simulink model "BB_DT_RRC_filters_EyeP_2020"  (R2020a)
settings: Solver=VariableStepDiscrete  StartTime=0.0  StopTime=L  RelTol=1e-3  AbsTol=1e-6  EnableMultiTasking=on
values from neighbouring files (symbols this model uses):
  G = 4    [ISI_init.m]
  N = 20    [ISI_init.m]
  R = 0.6    [ISI_init.m]
  T = 1e-3    (= 0.001)    [ISI_init.m]
undefined symbols (not defined in the file or in its folder): gcbh, rcfiltgaincompat
libraries: simulink_extras x9, commsequence2 x5, simulink x3, commfilt2 x2, commchan3 x1, dsparch4 x1
settings Model: Creator=calin  LastModifiedBy=Calin Vladeanu
settings DataIOCC: LimitDataPoints=on  SaveFormat=Array  SignalLoggingSaveFormat=ModelDataLogs  ReturnWorkspaceOutputs=off
settings OptimizationCC: InitFltsAndDblsToZero=on  LifeSpan=inf
settings DebuggingCC: SaveWithParameterizedLinksMsg=none  UnderspecifiedInitializationDetection=Classic  MergeDetectMultiDrivingBlocksExec=none  SignalResolutionControl=TryResolveAllWithWarning  SolverPrmCheckMsg=warning  MultiTaskDSMMsg=warning  MultiTaskCondExecSysMsg=none  FcnCallInpInsideContextMsg=warning  StateNameClashWarn=warning  SFUnexpectedBacktrackingDiag=warning  SFNoUnconditionalDefaultTransitionDiag=warning  SFExecutionAtInitializationDiag=none  ArithmeticOperatorsInVariantConditions=warning
settings HardwareCC: ProdBitPerPointer=32  ProdBitPerSizeT=32  ProdBitPerPtrDiffT=32  ProdLargestAtomicFloat=None  ProdIntDivRoundTo=Undefined  ProdEndianess=Unspecified  ProdWordSize=32  ProdHWDeviceType=32-bit Generic
settings ModelReferenceCC: PropagateSignalLabelsOutOfModel=off
settings SFSimCC: SimUseLocalCustomCode=off  CustomCodeUndefinedFunction=UseInterfaceOnly
settings RTWCC: RTWUseLocalCustomCode=off
settings CodeAppCC: StateflowObjectComments=on
settings GRTTargetCC: TargetFcnLib=ansi_tfl_tmw.mat  TargetLangStandard=C89/C90 (ANSI)  CombineOutputUpdateFcns=off  GRTInterface=on
settings ConfigComp: CovMetricSettings=dw  CovHtmlReporting=on  CovSaveCumulativeToWorkspaceVar=on  CovSaveSingleToWorkspaceVar=on  CovExternalEMLEnable=off

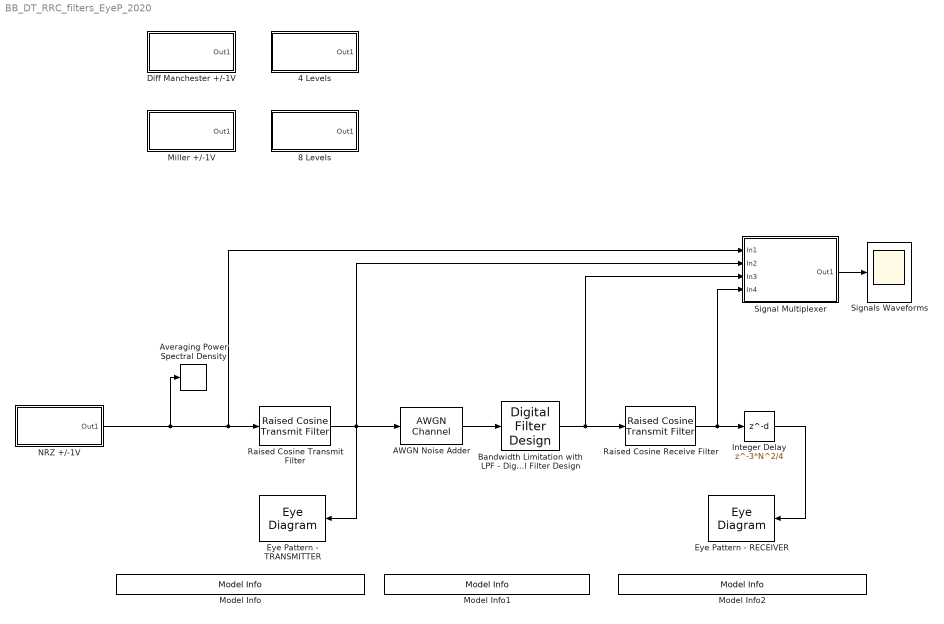
== system BB_DT_RRC_filters_EyeP_2020 ==
  4 Levels : Subsystem
  "8 Levels " : Subsystem
  AWGN Noise Adder : commchan3/AWGN Channel  InputProcessing=Columns as channels (frame based)  seed=67  noiseMode="Signal to noise ratio  (SNR)"  EbNodB=10  EsNodB=10  SNRdB=SNRdB  bitsPerSym=1  Ps=1  Tsym=1  variance=1
  Averaging Power Spectral Density : simulink_extras/Additional Sinks/Averaging Power Spectral Density  npts=512  fftpts=4096  HowOften=256  sampleT=T/8
      link override sfunpsd: FunctionName=sfunpsd_mod  Parameters=fftpts,npts,HowOften,offset,ts,1,type_disp
      settings: SourceProductBaseCode=SL
  Bandwidth Limitation with LPF - Digital Filter Design : dsparch4/Digital Filter Design  mwdsp_browser_bugfix_var=off
  Diff Manchester +/-1V : Subsystem
  Eye Pattern - RECEIVER : EyeDiagram  Tag=EyeDiagram
  Eye Pattern - TRANSMITTER : EyeDiagram  Tag=EyeDiagram
  Integer Delay : Delay  DelayLength=3*N^2/4
  Miller +/-1V : Subsystem
  Model Info : simulink/Model-Wide Utilities/Model Info  Frame=on  DisplayStringWithTags=TRANSMITTER  HorizontalTextAlignment=Center  LeftAlignmentValue=0.5
  Model Info1 : simulink/Model-Wide Utilities/Model Info  Frame=on  DisplayStringWithTags=CHANNEL MODEL  HorizontalTextAlignment=Center  LeftAlignmentValue=0.5
  Model Info2 : simulink/Model-Wide Utilities/Model Info  Frame=on  DisplayStringWithTags=RECEIVER  HorizontalTextAlignment=Center  LeftAlignmentValue=0.5
  NRZ +/-1V : Subsystem
  Raised Cosine Receive Filter : commfilt2/Raised Cosine Transmit Filter  filtType=Square root  R=R  filtSpan=2*(G)  N=N  filterGain=(sqrt(N))*rcfiltgaincompat(gcbh)  InputProcessing=Columns as channels (frame based)  RateOptions=Allow multirate processing  framing=Mute  checkCoeff=off  variableName=rcTxFilt1  checkGain=User-specified  sampMode=Mute  saveAsFlag=0  currentFiltSpan=2*(G)  D=G  launchFVT=off  roundingMode=Floor  overflowMode=off  coeffDataTypeStr=Inherit: Same word length as input  coeffMin=[]  coeffMax=[]  coeffLastDataTypeStr=Inherit: Same word length as input  outputDataTypeStr=Inherit: Same as accumulator  outputMin=[]  outputMax=[]  outputLastDataTypeStr=Inherit: Same as accumulator
  Raised Cosine Transmit Filter : commfilt2/Raised Cosine Transmit Filter  filtType=Square root  R=R  filtSpan=2*(G)  N=N  filterGain=(sqrt(N))*rcfiltgaincompat(gcbh)  InputProcessing=Columns as channels (frame based)  RateOptions=Allow multirate processing  framing=Mute  checkCoeff=off  variableName=rcTxFilt  checkGain=User-specified  sampMode=Mute  saveAsFlag=0  currentFiltSpan=2*(G)  D=G  launchFVT=off  roundingMode=Floor  overflowMode=off  coeffDataTypeStr=Inherit: Same word length as input  coeffMin=[]  coeffMax=[]  coeffLastDataTypeStr=Inherit: Same word length as input  outputDataTypeStr=Inherit: Same as accumulator  outputMin=[]  outputMax=[]  outputLastDataTypeStr=Inherit: Same as accumulator
  Signal Multiplexer : Subsystem
  Signals Waveforms : Scope
  wires:
  Raised Cosine Transmit Filter/1 -> AWGN Noise Adder/1, Eye Pattern - TRANSMITTER/1, Signal Multiplexer/2(In2)
  Raised Cosine Receive Filter/1 -> Integer Delay/1, Signal Multiplexer/4(In4)
  Bandwidth Limitation with LPF - Digital Filter Design/1 -> Raised Cosine Receive Filter/1, Signal Multiplexer/3(In3)
  AWGN Noise Adder/1 -> Bandwidth Limitation with LPF - Digital Filter Design/1
  Integer Delay/1 -> Eye Pattern - RECEIVER/1
  Signal Multiplexer/1(Out1) -> Signals Waveforms/1
  NRZ +/-1V/1(Out1) -> Averaging Power Spectral Density/1, Raised Cosine Transmit Filter/1, Signal Multiplexer/1(In1)

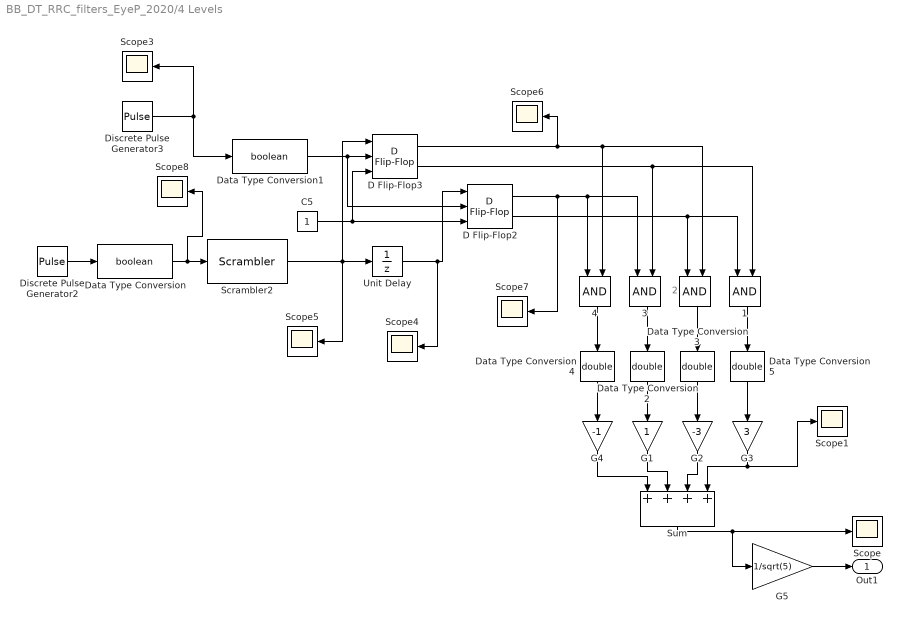
== system BB_DT_RRC_filters_EyeP_2020/4 Levels ==
  note: 2
  " " : Logic  OutDataTypeStr=boolean
  " 1" : Logic  OutDataTypeStr=boolean
  3 : Logic  OutDataTypeStr=boolean
  4 : Logic  OutDataTypeStr=boolean
  C5 : Constant
  D Flip-Flop2 : simulink_extras/Flip Flops/D Flip-Flop
  D Flip-Flop3 : simulink_extras/Flip Flops/D Flip-Flop
  Data Type Conversion : DataTypeConversion  OutDataTypeStr=boolean
  Data Type Conversion1 : DataTypeConversion  OutDataTypeStr=boolean
  Data Type Conversion{2..5} (4 alike) : DataTypeConversion  OutDataTypeStr=double
  Discrete Pulse Generator2 : DiscretePulseGenerator  Period=8  SampleTime=T
      settings: AttributesFormatString=1:7
  Discrete Pulse Generator3 : DiscretePulseGenerator  Period=4  PhaseDelay=2  SampleTime=T/2
      settings: AttributesFormatString=1:5
  G1 : Gain  OutDataTypeStr=double  SaturateOnIntegerOverflow=on  ParamDataTypeStr=Inherit: Same as input
  G2 : Gain  Gain=-3  OutDataTypeStr=double  SaturateOnIntegerOverflow=on  ParamDataTypeStr=Inherit: Same as input
  G3 : Gain  Gain=3  OutDataTypeStr=double  SaturateOnIntegerOverflow=on  ParamDataTypeStr=Inherit: Same as input
  G4 : Gain  Gain=-1  OutDataTypeStr=double  SaturateOnIntegerOverflow=on  ParamDataTypeStr=Inherit: Same as input
  G5 : Gain  Gain=1/sqrt(5)  OutDataTypeStr=double  SaturateOnIntegerOverflow=on  ParamDataTypeStr=Inherit: Same as input
  Scope{,1,3..8} (8 alike) : Scope
  Scrambler2 : commsequence2/Scrambler  M=2  poly=[0 -1 -7]  iniStaSource=Dialog Parameter  ini_sta=[1 1 1 1 1 1 1]  resetViaPort=off
      settings: SourceProductBaseCode=CM
  Sum : Sum  Inputs=++++  InputSameDT=on  AccumDataTypeStr=double  OutDataTypeStr=double  SaturateOnIntegerOverflow=on
  Unit Delay : UnitDelay  InitialCondition=1  SampleTime=-1  HasFrameUpgradeWarning=on
  Out1 : Outport  VectorParamsAs1DForOutWhenUnconnected=off
  wires:
  Sum/1 -> G5/1, Scope/1
  3/1 -> Data Type Conversion2/1
  " 1"/1 -> Data Type Conversion5/1
  D Flip-Flop2/1 -> 3/1, 4/1, Scope7/1
  D Flip-Flop2/2 -> " 1"/1, " "/1
  Scrambler2/1 -> D Flip-Flop3/1, Unit Delay/1, Scope5/1
  4/1 -> Data Type Conversion4/1
  C5/1 -> D Flip-Flop3/3, D Flip-Flop2/3
  Unit Delay/1 -> D Flip-Flop2/1, Scope4/1
  Discrete Pulse Generator2/1 -> Data Type Conversion/1
  D Flip-Flop3/1 -> " "/2, 4/2, Scope6/1
  " "/1 -> Data Type Conversion3/1
  D Flip-Flop3/2 -> " 1"/2, 3/2
  Discrete Pulse Generator3/1 -> Data Type Conversion1/1, Scope3/1
  Data Type Conversion/1 -> Scope8/1, Scrambler2/1
  Data Type Conversion1/1 -> D Flip-Flop3/2, D Flip-Flop2/2
  G4/1 -> Sum/1
  G1/1 -> Sum/2
  G2/1 -> Sum/3
  G3/1 -> Scope1/1, Sum/4
  Data Type Conversion4/1 -> G4/1
  Data Type Conversion2/1 -> G1/1
  Data Type Conversion3/1 -> G2/1
  Data Type Conversion5/1 -> G3/1
  G5/1 -> Out1/1

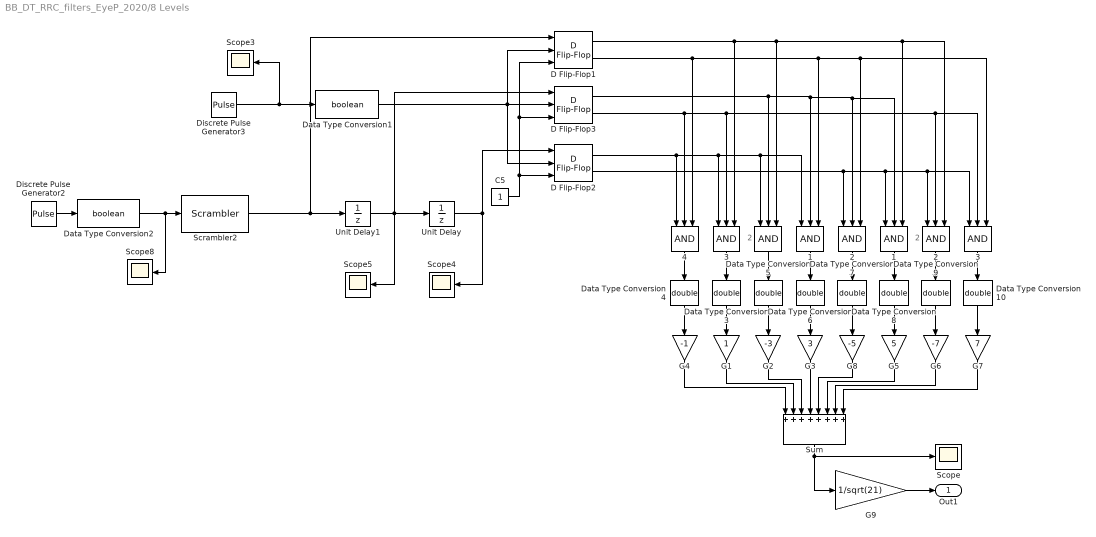
== system BB_DT_RRC_filters_EyeP_2020/8 Levels  ==
  note: 2
  note: 2
   {,1..3} (4 alike) : Logic  Inputs=3
  {1..4} (4 alike) : Logic  Inputs=3
  C5 : Constant
  D Flip-Flop1 : simulink_extras/Flip Flops/D Flip-Flop
  D Flip-Flop2 : simulink_extras/Flip Flops/D Flip-Flop
  D Flip-Flop3 : simulink_extras/Flip Flops/D Flip-Flop
  Data Type Conversion1 : DataTypeConversion  OutDataTypeStr=boolean
  Data Type Conversion{3..10} (8 alike) : DataTypeConversion  OutDataTypeStr=double
  Data Type Conversion2 : DataTypeConversion  OutDataTypeStr=boolean
  Discrete Pulse Generator2 : DiscretePulseGenerator  Period=8  SampleTime=2*pi/10000
      settings: AttributesFormatString=1:7
  Discrete Pulse Generator3 : DiscretePulseGenerator  Period=6  PhaseDelay=4  SampleTime=2*pi/20000
      settings: AttributesFormatString=1:5
  G1 : Gain  OutDataTypeStr=double  SaturateOnIntegerOverflow=on  ParamDataTypeStr=Inherit: Same as input
  G2 : Gain  Gain=-3  OutDataTypeStr=double  SaturateOnIntegerOverflow=on  ParamDataTypeStr=Inherit: Same as input
  G3 : Gain  Gain=3  OutDataTypeStr=double  SaturateOnIntegerOverflow=on  ParamDataTypeStr=Inherit: Same as input
  G4 : Gain  Gain=-1  OutDataTypeStr=double  SaturateOnIntegerOverflow=on  ParamDataTypeStr=Inherit: Same as input
  G5 : Gain  Gain=5  OutDataTypeStr=double  SaturateOnIntegerOverflow=on  ParamDataTypeStr=Inherit: Same as input
  G6 : Gain  Gain=-7  OutDataTypeStr=double  SaturateOnIntegerOverflow=on  ParamDataTypeStr=Inherit: Same as input
  G7 : Gain  Gain=7  OutDataTypeStr=double  SaturateOnIntegerOverflow=on  ParamDataTypeStr=Inherit: Same as input
  G8 : Gain  Gain=-5  OutDataTypeStr=double  SaturateOnIntegerOverflow=on  ParamDataTypeStr=Inherit: Same as input
  G9 : Gain  Gain=1/sqrt(21)  OutDataTypeStr=double  SaturateOnIntegerOverflow=on  ParamDataTypeStr=Inherit: Same as input
  Scope{,3..5,8} (5 alike) : Scope
  Scrambler2 : commsequence2/Scrambler  M=2  poly=[0 -1 -7]  iniStaSource=Dialog Parameter  ini_sta=[1 1 1 1 1 1 1]  resetViaPort=off
      settings: SourceProductBaseCode=CM
  Sum : Sum  Inputs=++++++++  InputSameDT=on  AccumDataTypeStr=double  OutDataTypeStr=double  SaturateOnIntegerOverflow=on
  Unit Delay : UnitDelay  InitialCondition=1  SampleTime=-1  HasFrameUpgradeWarning=on
  Unit Delay1 : UnitDelay  InitialCondition=1  SampleTime=-1  HasFrameUpgradeWarning=on
  Out1 : Outport  VectorParamsAs1DForOutWhenUnconnected=off
  wires:
  D Flip-Flop2/1 -> " 1"/1, " "/1, 3/1, 4/1
  D Flip-Flop3/1 -> 1/2, 2/2, " 1"/2, " "/2
  D Flip-Flop2/2 -> " 3"/1, " 2"/1, 1/1, 2/1
  G8/1 -> Sum/5
  " 2"/1 -> Data Type Conversion9/1
  G1/1 -> Sum/2
  D Flip-Flop1/2 -> " 3"/3, 2/3, " 1"/3, 4/3
  D Flip-Flop3/2 -> " 3"/2, " 2"/2, 3/2, 4/2
  " 1"/1 -> Data Type Conversion6/1
  " 3"/1 -> Data Type Conversion10/1
  3/1 -> Data Type Conversion3/1
  4/1 -> Data Type Conversion4/1
  " "/1 -> Data Type Conversion5/1
  G2/1 -> Sum/3
  2/1 -> Data Type Conversion7/1
  G7/1 -> Sum/8
  C5/1 -> D Flip-Flop1/3, D Flip-Flop3/3, D Flip-Flop2/3
  Discrete Pulse Generator2/1 -> Data Type Conversion2/1
  G3/1 -> Sum/4
  G6/1 -> Sum/7
  Unit Delay/1 -> D Flip-Flop2/1, Scope4/1
  G5/1 -> Sum/6
  Scrambler2/1 -> D Flip-Flop1/1, Unit Delay1/1
  G4/1 -> Sum/1
  D Flip-Flop1/1 -> " 2"/3, 1/3, " "/3, 3/3
  Unit Delay1/1 -> Unit Delay/1, Scope5/1, D Flip-Flop3/1
  Discrete Pulse Generator3/1 -> Data Type Conversion1/1, Scope3/1
  Sum/1 -> G9/1, Scope/1
  1/1 -> Data Type Conversion8/1
  Data Type Conversion1/1 -> D Flip-Flop2/2, D Flip-Flop3/2, D Flip-Flop1/2
  Data Type Conversion2/1 -> Scope8/1, Scrambler2/1
  Data Type Conversion4/1 -> G4/1
  Data Type Conversion3/1 -> G1/1
  Data Type Conversion5/1 -> G2/1
  Data Type Conversion6/1 -> G3/1
  Data Type Conversion7/1 -> G8/1
  Data Type Conversion8/1 -> G5/1
  Data Type Conversion9/1 -> G6/1
  Data Type Conversion10/1 -> G7/1
  G9/1 -> Out1/1

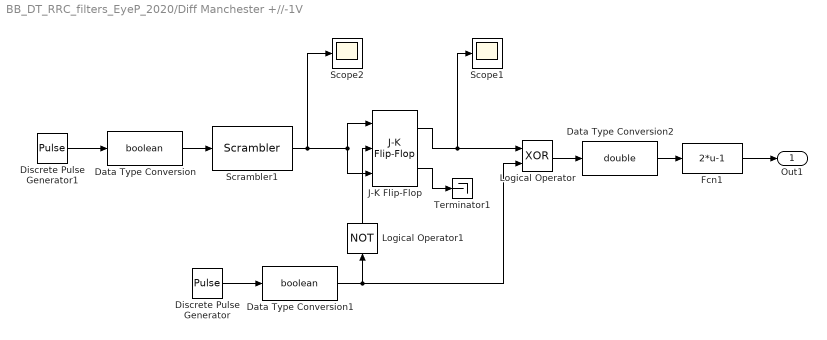
== system BB_DT_RRC_filters_EyeP_2020/Diff Manchester +//-1V ==
  Data Type Conversion : DataTypeConversion  OutDataTypeStr=boolean
  Data Type Conversion1 : DataTypeConversion  OutDataTypeStr=boolean
  Data Type Conversion2 : DataTypeConversion  OutDataTypeStr=double
  Discrete Pulse Generator : DiscretePulseGenerator  SampleTime=T/2
      settings: AttributesFormatString=CLK
  Discrete Pulse Generator1 : DiscretePulseGenerator  Period=8  SampleTime=T
      settings: AttributesFormatString=Data
  Fcn1 : Fcn  Expr=2*u-1
  J-K Flip-Flop : simulink_extras/Flip Flops/J-K Flip-Flop  initial_condition=0
  Logical Operator : Logic  Operator=XOR  OutDataTypeStr=boolean
  Logical Operator1 : Logic  Operator=NOT
  Scope1 : Scope
  Scope2 : Scope
  Scrambler1 : commsequence2/Scrambler  M=2  poly=[0 -1 -7]  iniStaSource=Dialog Parameter  ini_sta=[1 1 1 1 1 1 1]  resetViaPort=off
      settings: SourceProductBaseCode=CM
  Terminator1 : Terminator
  Out1 : Outport  VectorParamsAs1DForOutWhenUnconnected=off
  wires:
  Discrete Pulse Generator/1 -> Data Type Conversion1/1
  J-K Flip-Flop/2 -> Terminator1/1
  Logical Operator1/1 -> J-K Flip-Flop/2
  Scrambler1/1 -> Scope2/1, J-K Flip-Flop/1, J-K Flip-Flop/3
  Discrete Pulse Generator1/1 -> Data Type Conversion/1
  Logical Operator/1 -> Data Type Conversion2/1
  J-K Flip-Flop/1 -> Scope1/1, Logical Operator/1
  Data Type Conversion/1 -> Scrambler1/1
  Data Type Conversion1/1 -> Logical Operator1/1, Logical Operator/2
  Fcn1/1 -> Out1/1
  Data Type Conversion2/1 -> Fcn1/1

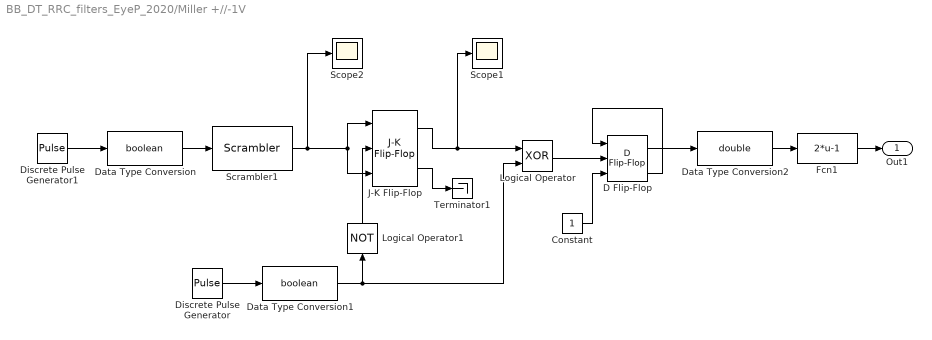
== system BB_DT_RRC_filters_EyeP_2020/Miller +//-1V ==
  Constant : Constant
  D Flip-Flop : simulink_extras/Flip Flops/D Flip-Flop
  Data Type Conversion : DataTypeConversion  OutDataTypeStr=boolean
  Data Type Conversion1 : DataTypeConversion  OutDataTypeStr=boolean
  Data Type Conversion2 : DataTypeConversion  OutDataTypeStr=double
  Discrete Pulse Generator : DiscretePulseGenerator  SampleTime=T/2
      settings: AttributesFormatString=CLK
  Discrete Pulse Generator1 : DiscretePulseGenerator  Period=8  SampleTime=T
      settings: AttributesFormatString=Data
  Fcn1 : Fcn  Expr=2*u-1
  J-K Flip-Flop : simulink_extras/Flip Flops/J-K Flip-Flop  initial_condition=0
  Logical Operator : Logic  Operator=XOR  OutDataTypeStr=boolean
  Logical Operator1 : Logic  Operator=NOT
  Scope1 : Scope
  Scope2 : Scope
  Scrambler1 : commsequence2/Scrambler  M=2  poly=[0 -1 -7]  iniStaSource=Dialog Parameter  ini_sta=[1 1 1 1 1 1 1]  resetViaPort=off
      settings: SourceProductBaseCode=CM
  Terminator1 : Terminator
  Out1 : Outport  VectorParamsAs1DForOutWhenUnconnected=off
  wires:
  Discrete Pulse Generator1/1 -> Data Type Conversion/1
  Data Type Conversion2/1 -> Fcn1/1
  Logical Operator/1 -> D Flip-Flop/2
  J-K Flip-Flop/2 -> Terminator1/1
  Scrambler1/1 -> Scope2/1, J-K Flip-Flop/1, J-K Flip-Flop/3
  Fcn1/1 -> Out1/1
  Data Type Conversion1/1 -> Logical Operator1/1, Logical Operator/2
  J-K Flip-Flop/1 -> Scope1/1, Logical Operator/1
  Discrete Pulse Generator/1 -> Data Type Conversion1/1
  Data Type Conversion/1 -> Scrambler1/1
  Logical Operator1/1 -> J-K Flip-Flop/2
  D Flip-Flop/2 -> D Flip-Flop/1
  Constant/1 -> D Flip-Flop/3
  D Flip-Flop/1 -> Data Type Conversion2/1

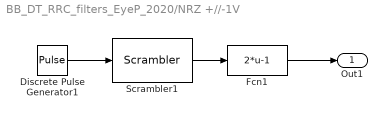
== system BB_DT_RRC_filters_EyeP_2020/NRZ +//-1V ==
  Discrete Pulse Generator1 : DiscretePulseGenerator  Period=8  SampleTime=T
      settings: AttributesFormatString=Data
  Fcn1 : Fcn  Expr=2*u-1
  Scrambler1 : commsequence2/Scrambler  M=2  poly=[0 -1 -7]  iniStaSource=Dialog Parameter  ini_sta=[1 1 1 1 1 1 1]  resetViaPort=off
      settings: SourceProductBaseCode=CM
  Out1 : Outport  VectorParamsAs1DForOutWhenUnconnected=off
  wires:
  Scrambler1/1 -> Fcn1/1
  Discrete Pulse Generator1/1 -> Scrambler1/1
  Fcn1/1 -> Out1/1

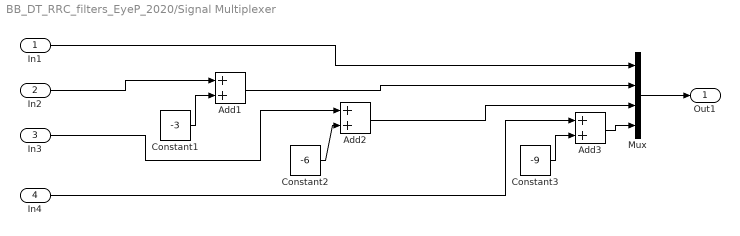
== system BB_DT_RRC_filters_EyeP_2020/Signal Multiplexer ==
  In1 : Inport
  In2 : Inport  Port=2
  In3 : Inport  Port=3
  In4 : Inport  Port=4
  Add1 : Sum
  Add2 : Sum
  Add3 : Sum
  Constant1 : Constant  Value=-3
  Constant2 : Constant  Value=-6
  Constant3 : Constant  Value=-9
  Mux : Mux
  Out1 : Outport  VectorParamsAs1DForOutWhenUnconnected=off
  wires:
  Mux/1 -> Out1/1
  Constant1/1 -> Add1/2
  Add1/1 -> Mux/2
  Constant2/1 -> Add2/2
  Add2/1 -> Mux/3
  Constant3/1 -> Add3/2
  Add3/1 -> Mux/4
  In1/1 -> Mux/1
  In2/1 -> Add1/1
  In3/1 -> Add2/1
  In4/1 -> Add3/1
